simulink model "simulator"  (R2014a)
settings: Solver=FixedStepDiscrete  StartTime=0.0  StopTime=80  FixedStep=0.01  RelTol=1e-3
PreLoadFcn:
  | VSS_RT_SYNC=Simulink.Variant('RT_SYNC==1');
  | RT_SYNC=0;
InitFcn:
  | load('buses/all_buses.mat');
  | load('scenario.mat');
StartFcn:
  | %clc;
  | addpath(strcat(fileparts(which(gcs)),'\figtitle'));
  | length=scenario.reference_command.Length;
  | te=str2num(get_param(gcs,'FixedStep'));
  | duration=(length-1)*te;
  | set_param(gcs,'StopTime',num2str(duration));
  | %variant_rt = Simulink.Variant('rt_sync==1');
StopFcn:
  | hws = get_param('simulator','modelworkspace');
  | plot_results = hws.getVariable('plot_results');
  | 
  | if(plot_results)
  |    f_plot_results;
  | end
model workspace (MAT data in the model file):
  incStep = 0.001
  decStep = 0.2
  decStepMax = 0.05
  plot_results = 1
  export_matfile = 0
  export_png = 0
values from neighbouring files (symbols this model uses):
  scenario = handles.scenario    [scenario_visualizer_gui.m]
libraries: my_library x8, rtwinlib x1
settings Model: ExtModeTrigDuration=100000  Creator=jean  LastModifiedBy=jean
settings DataIOCC: LimitDataPoints=off
settings OptimizationCC: OptimizeModelRefInitCode=on
settings HardwareCC: ProdIntDivRoundTo=Zero  ProdEndianess=LittleEndian  ProdHWDeviceType=Generic->32-bit x86 compatible
settings RTWCC: SystemTargetFile=rtwinert.tlc  TemplateMakefile=rtwinert.tmf  Description=Real-Time Windows Target (ERT)  ProcessScript=rtwinert_make_rtw_hook  RTWCompilerOptimization=On
settings CodeAppCC: MaxIdLength=95
settings RTWinTargetERTCC: TargetFcnLib=ansi_tfl_table_tmw.mat  TargetLibSuffix=_rtwin.lib  TargetPreCompLibLocation=C:\Program Files\MATLAB\R2014a\toolbox\rtw\targets\rtwin\lib\win64  GenFloatMathFcnCalls=NOT IN USE  TargetLangStandard=C89/C90 (ANSI)  CodeReplacementLibrary=None  UtilityFuncGeneration=Auto  ERTMultiwordTypeDef=System defined  ERTMultiwordLength=256  MultiwordLength=2048  GenerateFullHeader=on  GenerateSampleERTMain=off  GenerateTestInterfaces=off  ModelReferenceCompliant=on  ParMdlRefBuildCompliant=off  CompOptLevelCompliant=on  ConcurrentExecutionCompliant=off  IncludeMdlTerminateFcn=on  GeneratePreprocessorConditionals=Disable all  CombineOutputUpdateFcns=off  CombineSignalStateStructs=off  SuppressErrorStatus=off  ERTFirstTimeCompliant=off  IncludeFileDelimiter=Auto  ERTCustomFileBanners=off  SupportAbsoluteTime=on  LogVarNameModifier=rt_  MatFileLogging=off  MultiInstanceERTCode=off  CodeInterfacePackaging=Nonreusable function  SupportNonFinite=on  SupportComplex=on  PurelyIntegerCode=off  SupportContinuousTime=on  SupportNonInlinedSFcns=on  SupportVariableSizeSignals=on  EnableShiftOperators=on  ParenthesesLevel=Nominal  MATLABClassNameForMDSCustomization=Simulink.SoftwareTarget.TargetSpecificTriggerConfigurationBase  ModelStepFunctionPrototypeControlCompliant=off  CPPClassGenCompliant=off  AutosarCompliant=off  GRTInterface=off  GenerateAllocFcn=off  GenerateASAP2=off  InlinedParameterPlacement=NonHierarchical  TargetOS=BareBoardExample  MultiInstanceErrorCode=Error  RateGroupingCode=on  RootIOFormat=Individual arguments  RTWCAPISignals=off  RTWCAPIParams=off  RTWCAPIStates=off  RTWCAPIRootIO=off  ERTSrcFileBannerTemplate=ert_code_template.cgt  ERTHdrFileBannerTemplate=ert_code_template.cgt  ERTDataSrcFileTemplate=ert_code_template.cgt  ERTDataHdrFileTemplate=ert_code_template.cgt  ERTCustomFileTemplate=example_file_process.tlc  EnableDataOwnership=off  SignalDisplayLevel=10  ParamTuneLevel=10  GlobalDataDefinition=Auto  DataDefinitionFile=global.c  GlobalDataReference=Auto  ERTFilePackagingFormat=Modular  DataReferenceFile=global.h  PreserveExpressionOrder=off  PreserveIfCondition=off  ConvertIfToSwitch=off  PreserveExternInFcnDecls=on  SuppressUnreachableDefaultCases=off  IndentStyle=K&R  IndentSize=2  EnableUserReplacementTypes=off  MemSecPackage=--- None ---  MemSecDataConstants=Default  MemSecDataIO=Default  MemSecDataInternal=Default  MemSecDataParameters=Default  MemSecFuncInitTerm=Default  MemSecFuncExecute=Default  MemSecFuncSharedUtil=Default  CCListing=off  RebuildAll=off  ExtMode=on  ExtModeTransport=0  ExtModeStaticAlloc=off  ExtModeStaticAllocSize=1000000  ExtModeTesting=off  ExtModeMexFile=rtwinext  ExtModeIntrfLevel=Level1

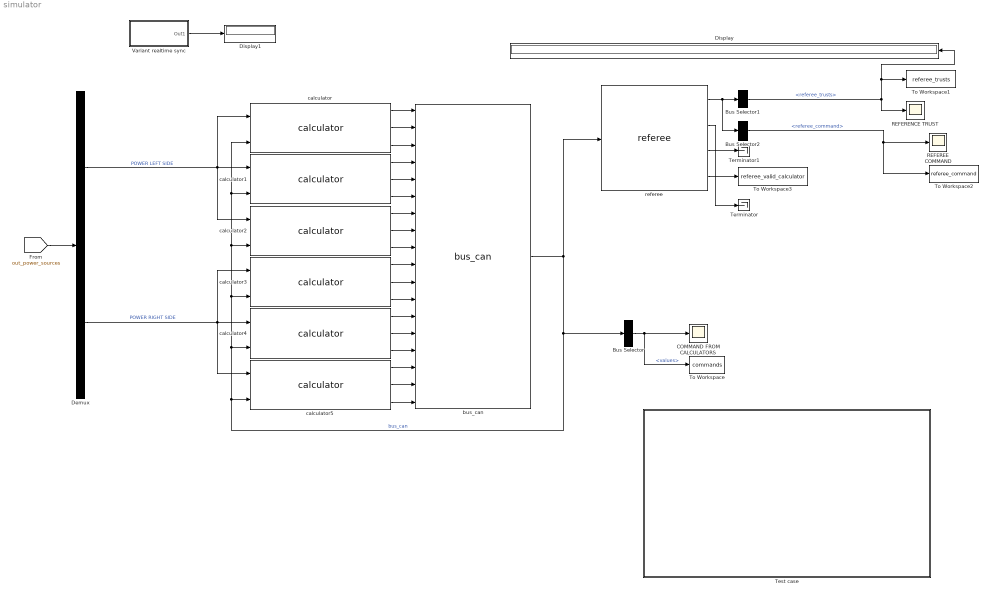
== system simulator ==
  Bus Selector : BusSelector  OutputSignals=calculators_outputs.calculators_commands.values
  Bus Selector1 : BusSelector  OutputSignals=referee_trusts
  Bus Selector2 : BusSelector  OutputSignals=referee_command
  COMMAND FROM CALCULATORS : Scope
      settings: YMin=2.5  YMax=7.75
  Demux : Demux  Outputs=2
  Display : Display
  Display1 : Display
  REFEREE COMMAND : Scope
      settings: YMin=2.25  YMax=6  SaveName=ScopeData2
  REFERENCE TRUST : Scope
      settings: TimeRange=10  YMin=-0.1  YMax=1.1
  Terminator : Terminator
  Terminator1 : Terminator
  Test case : Subsystem
      mask Display: image('images/writting_test_cases_in_software_testing_with_sample-1024x538.png');
  To Workspace : ToWorkspace  VariableName=commands  SaveFormat=Timeseries  SampleTime=-1
  To Workspace1 : ToWorkspace  VariableName=referee_trusts  SaveFormat=Timeseries  SampleTime=-1
  To Workspace2 : ToWorkspace  VariableName=referee_command  SaveFormat=Timeseries  SampleTime=-1
  To Workspace3 : ToWorkspace  VariableName=referee_valid_calculator  SaveFormat=Timeseries  SampleTime=-1
  Variant realtime sync : Subsystem  Variant=on
  bus_can : my_library/bus_can  SystemSampleTime=-1
  calculator : my_library/calculator  id=1
  calculator1 : my_library/calculator  id=2
  calculator2 : my_library/calculator  id=3
  calculator3 : my_library/calculator  id=4
  calculator4 : my_library/calculator  id=5
  calculator5 : my_library/calculator  id=6
  referee : my_library/referee  cmd_delay=3
  wires:
  Demux/1 -> calculator/1, calculator2/1, calculator1/1  "POWER LEFT SIDE"
  calculator/1 -> bus_can/1
  calculator/2 -> bus_can/2
  calculator/3 -> bus_can/3
  calculator1/2 -> bus_can/5
  calculator1/3 -> bus_can/6
  calculator1/1 -> bus_can/4
  calculator2/2 -> bus_can/8
  calculator2/3 -> bus_can/9
  calculator2/1 -> bus_can/7
  calculator3/3 -> bus_can/12
  calculator3/1 -> bus_can/10
  calculator3/2 -> bus_can/11
  calculator4/2 -> bus_can/14
  calculator4/1 -> bus_can/13
  calculator4/3 -> bus_can/15
  calculator5/1 -> bus_can/16
  calculator5/2 -> bus_can/17
  calculator5/3 -> bus_can/18
  Demux/2 -> calculator5/1, calculator3/1, calculator4/1  "POWER RIGHT SIDE"
  Bus Selector1/1 -> REFERENCE TRUST/1, To Workspace1/1, Display/1  "<referee_trusts>"
  Bus Selector2/1 -> REFEREE COMMAND/1, To Workspace2/1  "<referee_command>"
  bus_can/1 -> Bus Selector/1, calculator5/2, calculator4/2, calculator3/2, calculator2/2, calculator1/2, calculator/2, referee/1  "bus_can"
  [out_power_sources] -> Demux/1
  Variant realtime sync/1(Out1) -> Display1/1
  Bus Selector/1 -> COMMAND FROM CALCULATORS/1, To Workspace/1  "<values>"
  referee/1 -> Bus Selector2/1, Bus Selector1/1
  referee/4 -> To Workspace3/1
  referee/3 -> Terminator1/1
  referee/2 -> Terminator/1

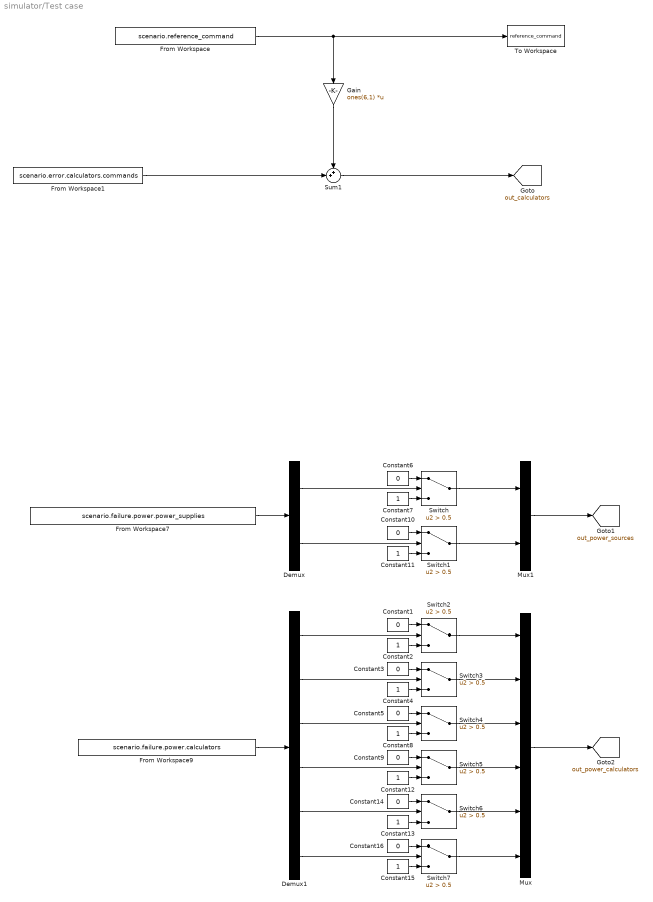
== system simulator/Test case ==
  Constant{1,3,5..6,9..10,14,16} (8 alike) : Constant  Value=0  OutDataTypeStr=uint8
  Constant{2,4,7..8,11..13,15} (8 alike) : Constant  OutDataTypeStr=uint8
  Demux : Demux  Outputs=2
  Demux1 : Demux  Outputs=6
  From Workspace : FromWorkspace  VariableName=scenario.reference_command  SampleTime=scenario.reference_command.Time(2)-scenario.reference_command.Time(1)  Interpolate=off  OutputAfterFinalValue=Setting to zero
  From Workspace1 : FromWorkspace  VariableName=scenario.error.calculators.commands  SampleTime=scenario.error.calculators.commands.Time(2)-scenario.error.calculators.commands.Time(1)  Interpolate=off  OutputAfterFinalValue=Setting to zero
  From Workspace7 : FromWorkspace  VariableName=scenario.failure.power.power_supplies  SampleTime=scenario.failure.power.power_supplies.Time(2)-scenario.failure.power.power_supplies.Time(1)
  From Workspace9 : FromWorkspace  VariableName=scenario.failure.power.calculators  SampleTime=scenario.failure.power.calculators.Time(2)-scenario.failure.power.calculators.Time(1)
  Gain : Gain  Gain=ones(6,1)  Multiplication=Matrix(K*u)
  Mux : Mux  Inputs=6
  Mux1 : Mux  Inputs=2
  Sum1 : Sum  Inputs=++|
  Switch{,1..7} (8 alike) : Switch  Criteria=u2 > Threshold  Threshold=0.5
  To Workspace : ToWorkspace  VariableName=reference_command  SaveFormat=Timeseries  SampleTime=-1
  tag scope: out_calculators=global, out_power_calculators=global, out_power_sources=global
  wires:
  From Workspace/1 -> Gain/1, To Workspace/1
  From Workspace1/1 -> Sum1/2
  Mux1/1 -> [out_power_sources]
  Constant6/1 -> Switch/1
  Constant7/1 -> Switch/3
  Constant10/1 -> Switch1/1
  Constant11/1 -> Switch1/3
  Demux/2 -> Switch1/2
  Switch/1 -> Mux1/1
  Switch1/1 -> Mux1/2
  Mux/1 -> [out_power_calculators]
  Constant1/1 -> Switch2/1
  Constant2/1 -> Switch2/3
  Switch2/1 -> Mux/1
  Constant3/1 -> Switch3/1
  Constant4/1 -> Switch3/3
  Constant5/1 -> Switch4/1
  Constant8/1 -> Switch4/3
  Constant9/1 -> Switch5/1
  Constant12/1 -> Switch5/3
  Constant14/1 -> Switch6/1
  Constant13/1 -> Switch6/3
  Constant16/1 -> Switch7/1
  Constant15/1 -> Switch7/3
  Demux1/2 -> Switch3/2
  Demux1/3 -> Switch4/2
  Demux1/4 -> Switch5/2
  Demux1/5 -> Switch6/2
  Demux1/6 -> Switch7/2
  Switch3/1 -> Mux/2
  Switch6/1 -> Mux/5
  Switch7/1 -> Mux/6
  Switch4/1 -> Mux/3
  Switch5/1 -> Mux/4
  Gain/1 -> Sum1/1
  Sum1/1 -> [out_calculators]
  Demux/1 -> Switch/2
  From Workspace7/1 -> Demux/1
  Demux1/1 -> Switch2/2
  From Workspace9/1 -> Demux1/1

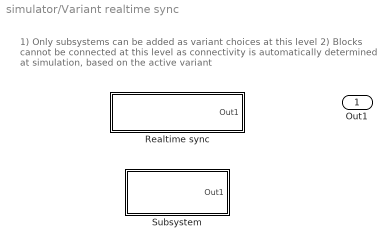
== system simulator/Variant realtime sync ==
  note: 1) Only subsystems can be added as variant choices at this level
      | 2) Blocks cannot be connected at this level as connectivity is
      | automatically determined at simulation, based on the active variant
  Realtime sync : Subsystem  VariantControl=VSS_RT_SYNC
  Subsystem : Subsystem  VariantControl=(default)
  Out1 : Outport

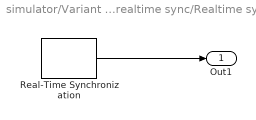
== system simulator/Variant realtime sync/Realtime sync ==
  Real-Time Synchronization : rtwinlib/Real-Time Synchronization  SampleTime=0.1  MaxMissedTicks=10  ShowMissedTicks=on  YieldWhenWaiting=off
  Out1 : Outport
  wires:
  Real-Time Synchronization/1 -> Out1/1

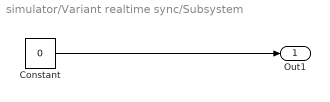
== system simulator/Variant realtime sync/Subsystem ==
  Constant : Constant  Value=0
  Out1 : Outport
  wires:
  Constant/1 -> Out1/1
